simulink model "New_Grashof"  (R2013b)
settings: Solver=FixedStepDiscrete  StartTime=0.0  StopTime=10  FixedStep=1  RelTol=1e-3
libraries: carnot x1
settings Model: Creator=awohlfei  LastModifiedBy=awohlfei
settings OptimizationCC: ExpressionDepthLimit=2147483647
settings DebuggingCC: UnderspecifiedInitializationDetection=Simplified  MergeDetectMultiDrivingBlocksExec=error  StateNameClashWarn=warning

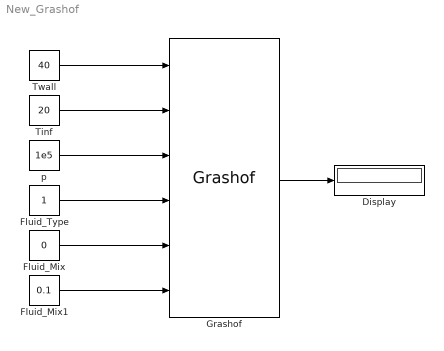
== system New_Grashof ==
  Display : Display
  Fluid_Mix : Constant  Value=0
  Fluid_Mix1 : Constant  Value=0.1
  Fluid_Type : Constant
  Grashof : carnot/Basic/Hydraulics/Grashof  VariantControl=CarlibClassic  DEBUGLEVEL=WARNINGLEVEL  MAXTOTALMESSAGES=inf  MAXCONSECUTIVEMESSAGES=inf  WRITETOFILE=0  FILENAME='errors.txt'
  Tinf : Constant  Value=20
  Twall : Constant  Value=40
  p : Constant  Value=1e5
  wires:
  Twall/1 -> Grashof/1
  p/1 -> Grashof/3
  Fluid_Type/1 -> Grashof/4
  Fluid_Mix/1 -> Grashof/5
  Grashof/1 -> Display/1
  Fluid_Mix1/1 -> Grashof/6
  Tinf/1 -> Grashof/2
